simulink model "line_following_2sensor"  (R2020a)
settings: Solver=VariableStepAuto  StartTime=0.0  StopTime=0.1  RelTol=1e-3
undefined symbols (not defined in the file or in its folder): duration, effort, index, joint_name, left_front, model_name, robotracer
libraries: robotgazebolib x6, simulink x1
settings Model: Creator=under  LastModifiedBy=under

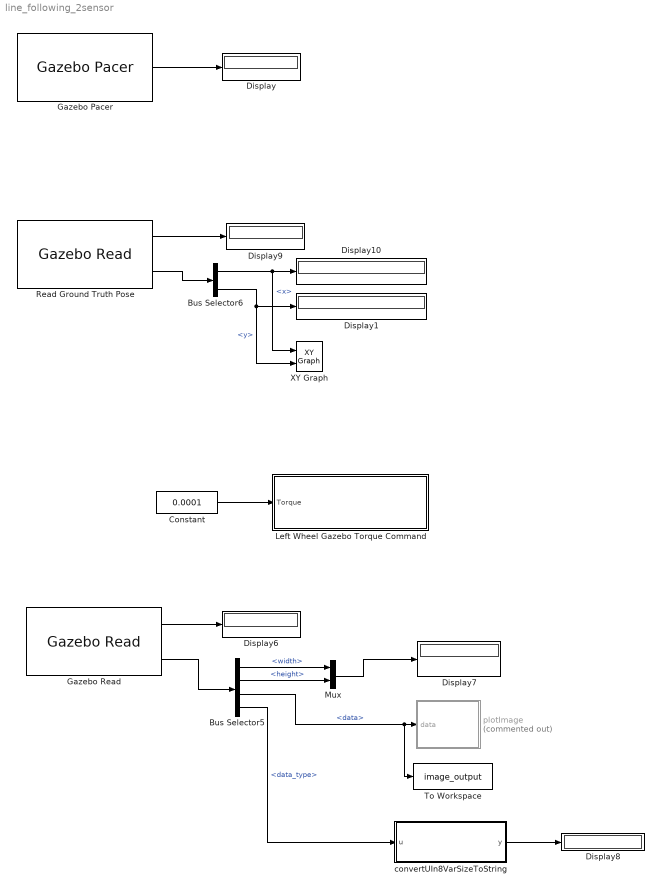
== system line_following_2sensor ==
  Bus Selector5 : BusSelector  OutputSignals=width,height,data,data_type
  Bus Selector6 : BusSelector  OutputSignals=position.x,position.y
  Constant : Constant  Value=0.0001
  Display{,1,6..10} (7 alike) : Display
  Gazebo Pacer : robotgazebolib/Gazebo Pacer  ResetBehavior=Reset Gazebo simulation time and scene  SampleTime=0.001
      settings: SourceProductBaseCode=RO
  Gazebo Read : robotgazebolib/Gazebo Read  topicSource=From Gazebo  topic=/gazebo/default/robotracer/camera2_link/camera2/image  messageType=gazebo_msgs/Image  sampleTime=0.001
      settings: SourceProductBaseCode=RO
  Left Wheel Gazebo Torque Command : Subsystem
  Mux : Mux  Inputs=2
  Read Ground Truth Pose : robotgazebolib/Gazebo Read  topicSource=From Gazebo  topic=/gazebo/ground_truth/world_pose/robotracer/chassis  messageType=gazebo_msgs/Pose  sampleTime=0.01
      settings: SourceProductBaseCode=RO
  To Workspace : ToWorkspace  VariableName=image_output  SaveFormat=Structure With Time  SampleTime=-1
  XY Graph : simulink/Sinks/XY Graph  xmin=-1  xmax=1  ymin=-1  ymax=1  st=-1
  convertUIn8VarSizeToString : MATLAB Function  TreatAsAtomicUnit=on
  plotImage : MATLAB Function  Commented=on  TreatAsAtomicUnit=on
  wires:
  Gazebo Pacer/1 -> Display/1
  Read Ground Truth Pose/2 -> Bus Selector6/1
  Bus Selector6/1 -> XY Graph/1, Display10/1  "<x>"
  Read Ground Truth Pose/1 -> Display9/1
  Bus Selector6/2 -> XY Graph/2, Display1/1  "<y>"
  Constant/1 -> Left Wheel Gazebo Torque Command/1(Torque)
  Gazebo Read/2 -> Bus Selector5/1
  Gazebo Read/1 -> Display6/1
  Bus Selector5/1 -> Mux/1  "<width>"
  Bus Selector5/2 -> Mux/2  "<height>"
  Mux/1 -> Display7/1
  Bus Selector5/3 -> To Workspace/1, plotImage/1(data)  "<data>"
  Bus Selector5/4 -> convertUIn8VarSizeToString/1(u)  "<data_type>"
  convertUIn8VarSizeToString/1(y) -> Display8/1

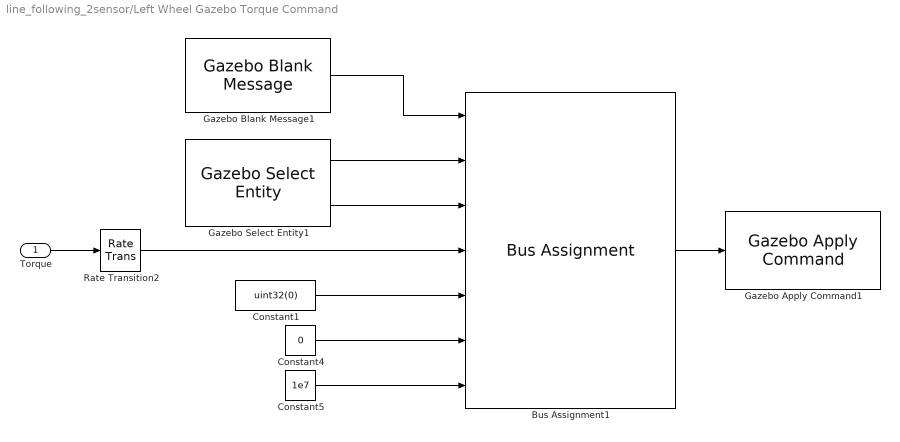
== system line_following_2sensor/Left Wheel Gazebo Torque Command ==
  Torque : Inport
  Bus Assignment1 : BusAssignment  AssignedSignals=model_name,joint_name,effort,index,duration.seconds,duration.nano_seconds
  Constant1 : Constant  Value=uint32(0)
  Constant4 : Constant  Value=0
  Constant5 : Constant  Value=1e7
  Gazebo Apply Command1 : robotgazebolib/Gazebo Apply Command  cmdType=ApplyJointTorque  sampleTime=0.01
      settings: SourceProductBaseCode=RO
  Gazebo Blank Message1 : robotgazebolib/Gazebo Blank Message  msgType=ApplyJointTorque  sampleTime=0.01  busName='Gazebo_SL_Bus_gazebo_msgs_ApplyJointTorque'
      settings: SourceProductBaseCode=RO
  Gazebo Select Entity1 : robotgazebolib/Gazebo Select Entity  modelElemName=robotracer/left_front  outputArraySize=128  OutputLabel=Joint  SelectType=Joint
      settings: SourceProductBaseCode=RO
  Rate Transition2 : RateTransition
  wires:
  Bus Assignment1/1 -> Gazebo Apply Command1/1
  Constant5/1 -> Bus Assignment1/7
  Gazebo Blank Message1/1 -> Bus Assignment1/1
  Gazebo Select Entity1/2 -> Bus Assignment1/3
  Gazebo Select Entity1/1 -> Bus Assignment1/2
  Torque/1 -> Rate Transition2/1
  Constant4/1 -> Bus Assignment1/6
  Rate Transition2/1 -> Bus Assignment1/4
  Constant1/1 -> Bus Assignment1/5

== matlab function line_following_2sensor/plotImage ==
  data: data input
function plotImage(data)

coder.extrinsic('imshow');
coder.extrinsic('helperPlotImage');

persistent h

if isempty(h)
    h = newplot(figure());
end


y = zeros(240, 320, 3, 'uint8');
if ~isempty(data) && ~isscalar(data)
    y(:) = helperPlotImage(data);
end
imshow(y, 'Parent', h);

== matlab function line_following_2sensor/convertUIn8VarSizeToString ==
  data: u input; y output string
function y = convertUInt8VarSizeToString(u)

y = convertCharsToStrings(char(u'));
